simulink model "exp_pos_servo_control_simu"  (R2020b)
settings: Solver=VariableStepAuto  StartTime=0.0  StopTime=tfinal  RelTol=1e-3
values from neighbouring files (symbols this model uses):
  A = [0,1;0,-1/T]    [exp_pos_state_control.m]    (also in pos_state_control.m; pos_state_control1.m)
  B = [0;K/T]    [exp_pos_state_control.m]    (also in pos_state_control.m; pos_state_control1.m)
  C = [1,0]    [exp_pos_state_control.m]    (also in pos_state_control.m; pos_state_control1.m)
  F = F_bar(1:2)    [exp_pos_state_control.m]    (also in pos_state_control.m)
  Ki = -F_bar(3)    [exp_pos_state_control.m]    (also in pos_state_control.m)
  r = 60    [exp_pos_state_control.m]    (also in pos_state_control.m; pos_state_control1.m)
  r_cyc = 8    [exp_pos_state_control.m]    (also in pos_state_control.m; pos_state_control1.m)
  ts = 1/50    (= 0.02)    [exp_pos_state_control.m]    (also in pos_state_control.m; pos_state_control1.m)
  x0 = [theta0;omega0]    [exp_pos_state_control.m]    (also in pos_state_control.m; pos_state_control1.m)
undefined symbols (not defined in the file or in its folder): DiscIntNeverNeededParam
libraries: arduino_io_lib x5
settings Model: Creator=kei55  LastModifiedBy=kei55

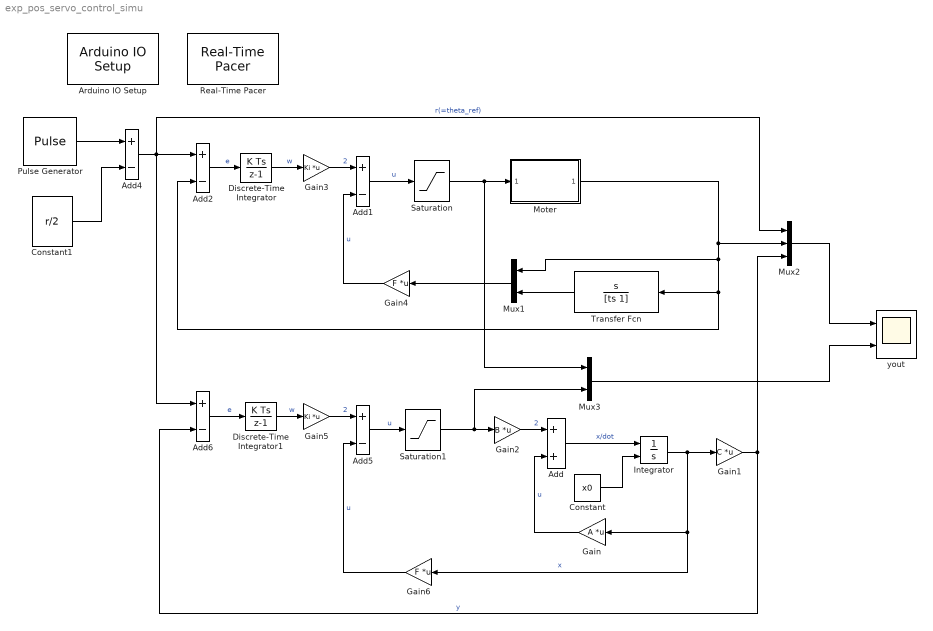
== system exp_pos_servo_control_simu ==
  Add : Sum
  Add{1..2,4..6} (5 alike) : Sum  Inputs=+-
  Arduino IO Setup : arduino_io_lib/Arduino IO Setup  Priority=3  arduinoVar=Temporary arduino variable: Arduino1  workspaceVarName=a  comPort=COM3
  Constant : Constant  Value=x0  VectorParams1D=off
  Constant1 : Constant  Value=r/2
  Discrete-Time Integrator : DiscreteIntegrator  SampleTime=ts  ICPrevOutput=DiscIntNeverNeededParam  ICPrevScaledInput=DiscIntNeverNeededParam
  Discrete-Time Integrator1 : DiscreteIntegrator  SampleTime=ts  ICPrevOutput=DiscIntNeverNeededParam  ICPrevScaledInput=DiscIntNeverNeededParam
  Gain : Gain  Gain=A  Multiplication=Matrix(K*u)
  Gain1 : Gain  Gain=C  Multiplication=Matrix(K*u)
  Gain2 : Gain  Gain=B  Multiplication=Matrix(K*u)
  Gain3 : Gain  Gain=Ki  Multiplication=Matrix(K*u)
  Gain4 : Gain  Gain=F  Multiplication=Matrix(K*u)
  Gain5 : Gain  Gain=Ki  Multiplication=Matrix(K*u)
  Gain6 : Gain  Gain=F  Multiplication=Matrix(K*u)
  Integrator : Integrator  InitialConditionSource=external
  Moter : Subsystem
  Mux1 : Mux  Inputs=2
  Mux2 : Mux  Inputs=3
  Mux3 : Mux  Inputs=2
  Pulse Generator : DiscretePulseGenerator  PulseType=Time based  Amplitude=r  Period=r_cyc  PulseWidth=50  SampleTime=1/50
  Real-Time Pacer : arduino_io_lib/Real-Time Pacer  simTimePerRealTime=1
  Saturation : Saturate  UpperLimit=5  LowerLimit=-5
  Saturation1 : Saturate  UpperLimit=5  LowerLimit=-5
  Transfer Fcn : TransferFcn  Numerator=[1 0]  Denominator=[ts 1]
  yout : Scope  NumInputPorts=2
  wires:
  Add/1 -> Integrator/1  "x/dot"
  Integrator/1 -> Gain1/1, Gain/1, Gain6/1  "x"
  Gain2/1 -> Add/1  "2"
  Gain/1 -> Add/2  "u"
  Constant/1 -> Integrator/2
  Gain3/1 -> Add1/1  "2"
  Add4/1 -> Mux2/1, Add2/1, Add6/1  "r(=theta_ref)"
  Gain4/1 -> Add1/2  "u"
  Constant1/1 -> Add4/2
  Pulse Generator/1 -> Add4/1
  Discrete-Time Integrator/1 -> Gain3/1  "w"
  Add1/1 -> Saturation/1  "u"
  Saturation/1 -> Mux3/1, Moter/1(va input)
  Mux1/1 -> Gain4/1
  Moter/1(theta pot) -> Mux1/1, Add2/2, Transfer Fcn/1, Mux2/2
  Add5/1 -> Saturation1/1  "u"
  Discrete-Time Integrator1/1 -> Gain5/1  "w"
  Gain6/1 -> Add5/2  "u"
  Gain5/1 -> Add5/1  "2"
  Saturation1/1 -> Mux3/2, Gain2/1
  Gain1/1 -> Add6/2, Mux2/3  "y"
  Mux3/1 -> yout/2
  Mux2/1 -> yout/1
  Add2/1 -> Discrete-Time Integrator/1  "e"
  Add6/1 -> Discrete-Time Integrator1/1  "e"
  Transfer Fcn/1 -> Mux1/2

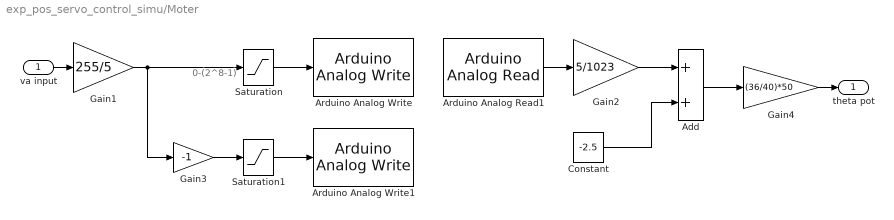
== system exp_pos_servo_control_simu/Moter ==
  note: 0-(2^8-1)
  va input : Inport
  Add : Sum
  Arduino Analog Read1 : arduino_io_lib/Arduino Analog Read  arduinoVar=Temporary arduino variable: Arduino1  arduinoPin=0  T=1/50
  Arduino Analog Write : arduino_io_lib/Arduino Analog Write  arduinoVar=Temporary arduino variable: Arduino1  arduinoPin=3  T=1/50
  Arduino Analog Write1 : arduino_io_lib/Arduino Analog Write  arduinoVar=Temporary arduino variable: Arduino1  arduinoPin=5  T=1/50
  Constant : Constant  Value=-2.5
  Gain1 : Gain  Gain=255/5
  Gain2 : Gain  Gain=5/1023
  Gain3 : Gain  Gain=-1
  Gain4 : Gain  Gain=(36/40)*50
  Saturation : Saturate  UpperLimit=255  LowerLimit=0
  Saturation1 : Saturate  UpperLimit=255  LowerLimit=0
  theta pot : Outport
  wires:
  Add/1 -> Gain4/1
  Constant/1 -> Add/2
  Gain2/1 -> Add/1
  Gain4/1 -> theta pot/1
  Gain3/1 -> Saturation1/1
  Gain1/1 -> Saturation/1, Gain3/1
  Saturation1/1 -> Arduino Analog Write1/1
  Saturation/1 -> Arduino Analog Write/1
  va input/1 -> Gain1/1
  Arduino Analog Read1/1 -> Gain2/1
